simulink model "StereoTypeRobot"  (R2024a)
settings: Solver=VariableStepAuto  StartTime=0.0  StopTime=10.0  RelTol=1e-3
settings Model: Creator=Tamir Azaouag  LastModifiedBy=Tamir Azaouag

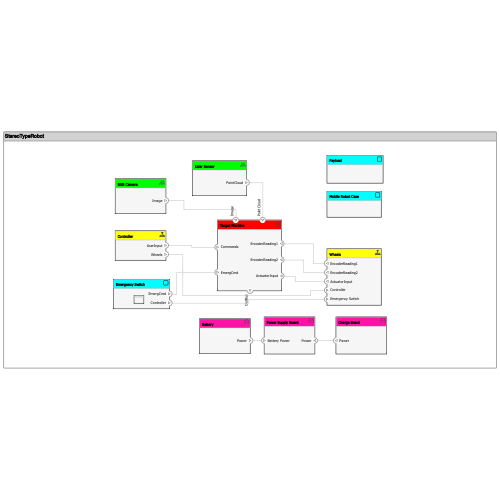
[thumbnail: Simulink's stored preview of the top-level diagram]
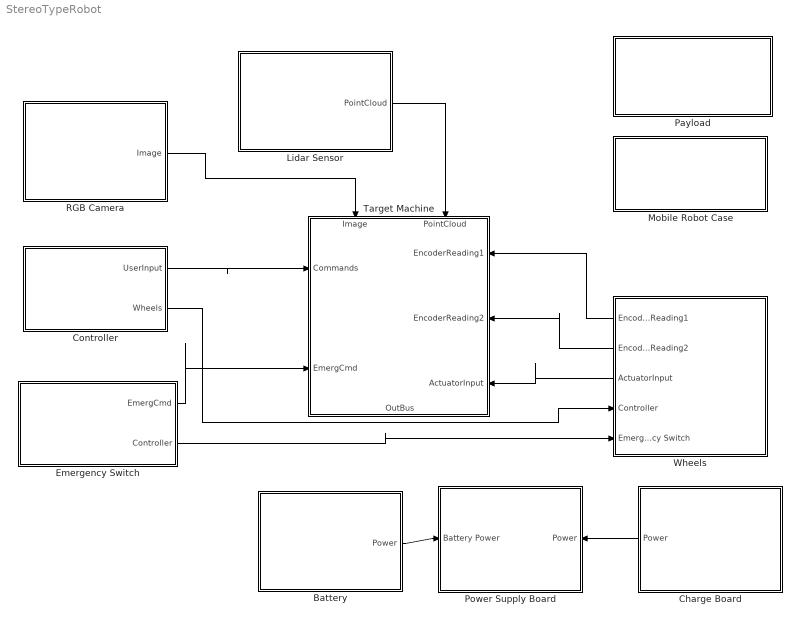
== system StereoTypeRobot ==
  "Battery " : Subsystem
      settings: PortSchema="{\"entries\":[{\"content\":{\"headerSize\":26,\"margin\":15,\"minimumSpacing\":25,\"sides\":[{\"content\":{},\"type\":\"ConnectorPlacement.EquallySpacedRectSide\",\"uuid\":\"52cfc6e8-b07b-405a-8482-438c255d2b0b\"},{\"content\":{\"connectorIds\":[\"Out1\"],\"side\":\"RIGHT\"},\"type\":\"ConnectorPlacement.EquallySpacedRectSide\",\"uuid\":\"f1465f6c-6812-4300-a41b-f67868e7a52d\"},{\"content\":{\"side\":\"TOP\"},\"type\":\"ConnectorPlacement.EquallySpacedRectSide\",\"uuid\":\"9b9722d7-8bd9-4c61-a011-ea6ff4bfa1dc\"}]},\"type\":\"ConnectorPlacement.EquallySpacedConnector\",\"uuid\":\"a33ceaa1-2646-464b-956e-0a789ac4e4be\"}],\"packageUris\":[\"http://schema.mathworks.com/mf0/Connector/R2020b\"],\"version\":\"1.0\"}"
  Charge Board : Subsystem
      settings: PortSchema="{\"entries\":[{\"content\":{\"headerSize\":26,\"margin\":15,\"minimumSpacing\":25,\"sides\":[{\"content\":{\"connectorIds\":[\"Out1\"]},\"type\":\"ConnectorPlacement.EquallySpacedRectSide\",\"uuid\":\"52cfc6e8-b07b-405a-8482-438c255d2b0b\"},{\"content\":{\"side\":\"RIGHT\"},\"type\":\"ConnectorPlacement.EquallySpacedRectSide\",\"uuid\":\"f1465f6c-6812-4300-a41b-f67868e7a52d\"},{\"content\":{\"side\":\"TOP\"},\"type\":\"ConnectorPlacement.EquallySpacedRectSide\",\"uuid\":\"9b9722d7-8bd9-4c61-a011-ea6ff4bfa1dc\"},{\"content\":{\"side\":\"BOTTOM\"},\"type\":\"ConnectorPlacement.EquallySpacedRectSide\",\"uuid\":\"8ae938ba-d761-47b8-bf48-a696c12dfec8\"}]},\"type\":\"ConnectorPlacement.EquallySpacedConnector\",\"uuid\":\"a33ceaa1-2646-464b-956e-0a789ac4e4be\"}],\"packageUris\":[\"http://schema.mathworks.com/mf0/Connector/R2020b\"],\"version\":\"1.0\"}"
  Controller : Subsystem
      settings: PortSchema="{\"entries\":[{\"content\":{\"headerSize\":26,\"margin\":15,\"minimumSpacing\":25,\"sides\":[{\"content\":{},\"type\":\"ConnectorPlacement.EquallySpacedRectSide\",\"uuid\":\"52cfc6e8-b07b-405a-8482-438c255d2b0b\"},{\"content\":{\"connectorIds\":[\"Out1\",\"Out2\"],\"side\":\"RIGHT\"},\"type\":\"ConnectorPlacement.EquallySpacedRectSide\",\"uuid\":\"f1465f6c-6812-4300-a41b-f67868e7a52d\"},{\"content\":{\"side\":\"TOP\"},\"type\":\"ConnectorPlacement.EquallySpacedRectSide\",\"uuid\":\"9b9722d7-8bd9-4c61-a011-ea6ff4bfa1dc\"}]},\"type\":\"ConnectorPlacement.EquallySpacedConnector\",\"uuid\":\"a33ceaa1-2646-464b-956e-0a789ac4e4be\"}],\"packageUris\":[\"http://schema.mathworks.com/mf0/Connector/R2020b\"],\"version\":\"1.0\"}"
  "Emergency Switch " : Subsystem
      settings: PortSchema="{\"entries\":[{\"content\":{\"headerSize\":26,\"margin\":15,\"minimumSpacing\":25,\"sides\":[{\"content\":{},\"type\":\"ConnectorPlacement.EquallySpacedRectSide\",\"uuid\":\"52cfc6e8-b07b-405a-8482-438c255d2b0b\"},{\"content\":{\"connectorIds\":[\"Out1\",\"Out2\"],\"side\":\"RIGHT\"},\"type\":\"ConnectorPlacement.EquallySpacedRectSide\",\"uuid\":\"f1465f6c-6812-4300-a41b-f67868e7a52d\"},{\"content\":{\"side\":\"TOP\"},\"type\":\"ConnectorPlacement.EquallySpacedRectSide\",\"uuid\":\"9b9722d7-8bd9-4c61-a011-ea6ff4bfa1dc\"}]},\"type\":\"ConnectorPlacement.EquallySpacedConnector\",\"uuid\":\"a33ceaa1-2646-464b-956e-0a789ac4e4be\"}],\"packageUris\":[\"http://schema.mathworks.com/mf0/Connector/R2020b\"],\"version\":\"1.0\"}"
  Lidar Sensor : Subsystem
      settings: PortSchema="{\"entries\":[{\"content\":{\"headerSize\":26,\"margin\":15,\"minimumSpacing\":25,\"sides\":[{\"content\":{},\"type\":\"ConnectorPlacement.EquallySpacedRectSide\",\"uuid\":\"52cfc6e8-b07b-405a-8482-438c255d2b0b\"},{\"content\":{\"connectorIds\":[\"Out1\"],\"side\":\"RIGHT\"},\"type\":\"ConnectorPlacement.EquallySpacedRectSide\",\"uuid\":\"f1465f6c-6812-4300-a41b-f67868e7a52d\"},{\"content\":{\"side\":\"TOP\"},\"type\":\"ConnectorPlacement.EquallySpacedRectSide\",\"uuid\":\"9b9722d7-8bd9-4c61-a011-ea6ff4bfa1dc\"}]},\"type\":\"ConnectorPlacement.EquallySpacedConnector\",\"uuid\":\"a33ceaa1-2646-464b-956e-0a789ac4e4be\"}],\"packageUris\":[\"http://schema.mathworks.com/mf0/Connector/R2020b\"],\"version\":\"1.0\"}"
  Mobile Robot Case : Subsystem
      settings: PortSchema="{\"entries\":[{\"content\":{\"headerSize\":26,\"margin\":15,\"minimumSpacing\":25,\"sides\":[{\"content\":{},\"type\":\"ConnectorPlacement.EquallySpacedRectSide\",\"uuid\":\"52cfc6e8-b07b-405a-8482-438c255d2b0b\"},{\"content\":{\"side\":\"RIGHT\"},\"type\":\"ConnectorPlacement.EquallySpacedRectSide\",\"uuid\":\"f1465f6c-6812-4300-a41b-f67868e7a52d\"},{\"content\":{\"side\":\"TOP\"},\"type\":\"ConnectorPlacement.EquallySpacedRectSide\",\"uuid\":\"9b9722d7-8bd9-4c61-a011-ea6ff4bfa1dc\"}]},\"type\":\"ConnectorPlacement.EquallySpacedConnector\",\"uuid\":\"a33ceaa1-2646-464b-956e-0a789ac4e4be\"}],\"packageUris\":[\"http://schema.mathworks.com/mf0/Connector/R2020b\"],\"version\":\"1.0\"}"
  Payload : Subsystem
      settings: PortSchema="{\"entries\":[{\"content\":{\"headerSize\":26,\"margin\":15,\"minimumSpacing\":25,\"sides\":[{\"content\":{},\"type\":\"ConnectorPlacement.EquallySpacedRectSide\",\"uuid\":\"52cfc6e8-b07b-405a-8482-438c255d2b0b\"},{\"content\":{\"side\":\"RIGHT\"},\"type\":\"ConnectorPlacement.EquallySpacedRectSide\",\"uuid\":\"f1465f6c-6812-4300-a41b-f67868e7a52d\"},{\"content\":{\"side\":\"TOP\"},\"type\":\"ConnectorPlacement.EquallySpacedRectSide\",\"uuid\":\"9b9722d7-8bd9-4c61-a011-ea6ff4bfa1dc\"}]},\"type\":\"ConnectorPlacement.EquallySpacedConnector\",\"uuid\":\"a33ceaa1-2646-464b-956e-0a789ac4e4be\"}],\"packageUris\":[\"http://schema.mathworks.com/mf0/Connector/R2020b\"],\"version\":\"1.0\"}"
  Power Supply Board : Subsystem
      settings: PortSchema="{\"entries\":[{\"content\":{\"headerSize\":26,\"margin\":15,\"minimumSpacing\":25,\"sides\":[{\"content\":{\"connectorIds\":[\"In2\"]},\"type\":\"ConnectorPlacement.EquallySpacedRectSide\",\"uuid\":\"52cfc6e8-b07b-405a-8482-438c255d2b0b\"},{\"content\":{\"connectorIds\":[\"In1\"],\"side\":\"RIGHT\"},\"type\":\"ConnectorPlacement.EquallySpacedRectSide\",\"uuid\":\"f1465f6c-6812-4300-a41b-f67868e7a52d\"},{\"content\":{\"side\":\"TOP\"},\"type\":\"ConnectorPlacement.EquallySpacedRectSide\",\"uuid\":\"9b9722d7-8bd9-4c61-a011-ea6ff4bfa1dc\"}]},\"type\":\"ConnectorPlacement.EquallySpacedConnector\",\"uuid\":\"a33ceaa1-2646-464b-956e-0a789ac4e4be\"}],\"packageUris\":[\"http://schema.mathworks.com/mf0/Connector/R2020b\"],\"version\":\"1.0\"}"
  RGB Camera : Subsystem
      settings: PortSchema="{\"entries\":[{\"content\":{\"headerSize\":26,\"margin\":15,\"minimumSpacing\":25,\"sides\":[{\"content\":{},\"type\":\"ConnectorPlacement.EquallySpacedRectSide\",\"uuid\":\"52cfc6e8-b07b-405a-8482-438c255d2b0b\"},{\"content\":{\"connectorIds\":[\"Out1\"],\"side\":\"RIGHT\"},\"type\":\"ConnectorPlacement.EquallySpacedRectSide\",\"uuid\":\"f1465f6c-6812-4300-a41b-f67868e7a52d\"},{\"content\":{\"side\":\"TOP\"},\"type\":\"ConnectorPlacement.EquallySpacedRectSide\",\"uuid\":\"9b9722d7-8bd9-4c61-a011-ea6ff4bfa1dc\"},{\"content\":{\"side\":\"BOTTOM\"},\"type\":\"ConnectorPlacement.EquallySpacedRectSide\",\"uuid\":\"a62c9273-1260-4d0a-a60b-7323b4ab9545\"}]},\"type\":\"ConnectorPlacement.EquallySpacedConnector\",\"uuid\":\"a33ceaa1-2646-464b-956e-0a789ac4e4be\"}],\"packageUris\":[\"http://schema.mathworks.com/mf0/Connector/R2020b\"],\"version\":\"1.0\"}"
  Target Machine : Subsystem
      settings: PortSchema="{\"entries\":[{\"content\":{\"headerSize\":26,\"margin\":15,\"minimumSpacing\":25,\"sides\":[{\"content\":{\"connectorIds\":[\"In6\",\"In7\"]},\"type\":\"ConnectorPlacement.EquallySpacedRectSide\",\"uuid\":\"52cfc6e8-b07b-405a-8482-438c255d2b0b\"},{\"content\":{\"connectorIds\":[\"In1\",\"In2\",\"In3\"],\"side\":\"RIGHT\"},\"type\":\"ConnectorPlacement.EquallySpacedRectSide\",\"uuid\":\"f1465f6c-6812-4300-a41b-f67868e7a52d\"},{\"content\":{\"connectorIds\":[\"In4\",\"In5\"],\"side\":\"TOP\"},\"type\":\"ConnectorPlacement.EquallySpacedRectSide\",\"uuid\":\"9b9722d7-8bd9-4c61-a011-ea6ff4bfa1dc\"},{\"content\":{\"connectorIds\":[\"Out1\"],\"side\":\"BOTTOM\"},\"type\":\"ConnectorPlacement.EquallySpacedRectSide\",\"uuid\":\"d37188e4-ada9-42bd-a53b-1c1899413b13\"}]},\"type\":\"ConnectorPlacement.EquallySpacedConnector\",\"uuid\":\"a33ceaa1-2646-464b-956e-0a789ac4e4be\"}],\"packageUris\":[\"http://schema.mathworks.com/mf0/Connector/R2020b\"],\"version\":\"1.0\"}"
  Wheels : Subsystem
      settings: PortSchema="{\"entries\":[{\"content\":{\"headerSize\":26,\"margin\":15,\"minimumSpacing\":25,\"sides\":[{\"content\":{\"connectorIds\":[\"Out3\",\"Out2\",\"Out1\",\"In1\",\"In2\"]},\"type\":\"ConnectorPlacement.EquallySpacedRectSide\",\"uuid\":\"52cfc6e8-b07b-405a-8482-438c255d2b0b\"},{\"content\":{\"side\":\"RIGHT\"},\"type\":\"ConnectorPlacement.EquallySpacedRectSide\",\"uuid\":\"f1465f6c-6812-4300-a41b-f67868e7a52d\"},{\"content\":{\"side\":\"TOP\"},\"type\":\"ConnectorPlacement.EquallySpacedRectSide\",\"uuid\":\"9b9722d7-8bd9-4c61-a011-ea6ff4bfa1dc\"},{\"content\":{\"side\":\"BOTTOM\"},\"type\":\"ConnectorPlacement.EquallySpacedRectSide\",\"uuid\":\"b29c40a7-1ea8-42d5-9ecb-a2e658638a42\"}]},\"type\":\"ConnectorPlacement.EquallySpacedConnector\",\"uuid\":\"a33ceaa1-2646-464b-956e-0a789ac4e4be\"}],\"packageUris\":[\"http://schema.mathworks.com/mf0/Connector/R2020b\"],\"version\":\"1.0\"}"
  wires:
  "Emergency Switch "/1(EmergCmd) -> Target Machine/7(EmergCmd)
  Controller/1(UserInput) -> Target Machine/6(Commands)
  RGB Camera/1(Image) -> Target Machine/4(Image)
  Lidar Sensor/1(PointCloud) -> Target Machine/5(PointCloud)
  "Battery "/1(Power) -> Power Supply Board/2(Battery Power)
  Charge Board/1(Power) -> Power Supply Board/1(Power)
  Wheels/3(EncoderReading1) -> Target Machine/1(EncoderReading1)
  Wheels/2(EncoderReading2) -> Target Machine/2(EncoderReading2)
  Wheels/1(ActuatorInput) -> Target Machine/3(ActuatorInput)
  Controller/2(Wheels) -> Wheels/1(Controller)
  "Emergency Switch "/2(Controller) -> Wheels/2("Emergency Switch ")

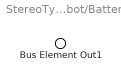
== system StereoTypeRobot/Battery  ==
  Bus Element Out1 : Outport  PortName=Power

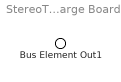
== system StereoTypeRobot/Charge Board ==
  Bus Element Out1 : Outport  PortName=Power

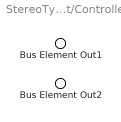
== system StereoTypeRobot/Controller ==
  Bus Element Out1 : Outport  PortName=UserInput
  Bus Element Out2 : Outport  Port=2  PortName=Wheels

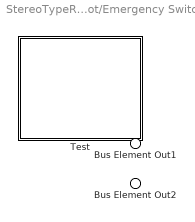
== system StereoTypeRobot/Emergency Switch  ==
  Test : Subsystem
      settings: PortSchema="{\"entries\":[{\"content\":{\"headerSize\":26,\"margin\":15,\"minimumSpacing\":25,\"sides\":[{\"content\":{},\"type\":\"ConnectorPlacement.EquallySpacedRectSide\",\"uuid\":\"a14bca50-eec3-4643-9852-5ab0485d1fad\"},{\"content\":{\"side\":\"RIGHT\"},\"type\":\"ConnectorPlacement.EquallySpacedRectSide\",\"uuid\":\"4c9be622-01ab-4851-b0cd-6570d8f0c0ef\"},{\"content\":{\"side\":\"TOP\"},\"type\":\"ConnectorPlacement.EquallySpacedRectSide\",\"uuid\":\"0b0c369c-b5bb-4b7a-9b2a-cb3d1555d7c6\"}]},\"type\":\"ConnectorPlacement.EquallySpacedConnector\",\"uuid\":\"40fee69b-64dd-44a3-a56b-f30c2048f046\"}],\"packageUris\":[\"http://schema.mathworks.com/mf0/Connector/R2020b\"],\"version\":\"1.0\"}"
  Bus Element Out1 : Outport  PortName=EmergCmd
  Bus Element Out2 : Outport  Port=2  PortName=Controller

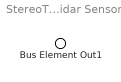
== system StereoTypeRobot/Lidar Sensor ==
  Bus Element Out1 : Outport  PortName=PointCloud

== system StereoTypeRobot/Mobile Robot Case ==

== system StereoTypeRobot/Payload ==

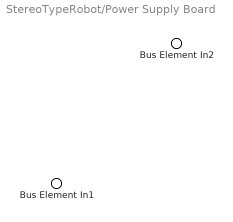
== system StereoTypeRobot/Power Supply Board ==
  Bus Element In2 : Inport  PortName=Power
  Bus Element In1 : Inport  Port=2  PortName=Battery Power

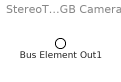
== system StereoTypeRobot/RGB Camera ==
  Bus Element Out1 : Outport  PortName=Image

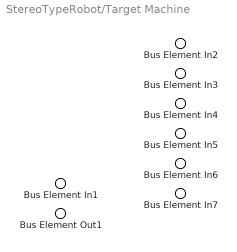
== system StereoTypeRobot/Target Machine ==
  Bus Element In5 : Inport  PortName=EncoderReading1
  Bus Element In6 : Inport  Port=2  PortName=EncoderReading2
  Bus Element In7 : Inport  Port=3  PortName=ActuatorInput
  Bus Element In3 : Inport  Port=4  PortName=Image
  Bus Element In4 : Inport  Port=5  PortName=PointCloud
  Bus Element In2 : Inport  Port=6  PortName=Commands
  Bus Element In1 : Inport  Port=7  PortName=EmergCmd
  Bus Element Out1 : Outport  PortName=OutBus

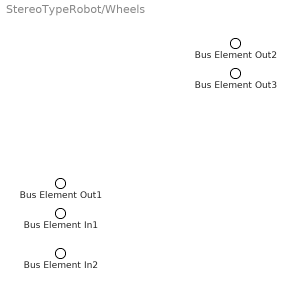
== system StereoTypeRobot/Wheels ==
  Bus Element In1 : Inport  PortName=Controller
  Bus Element In2 : Inport  Port=2  PortName=Emergency Switch
  Bus Element Out3 : Outport  PortName=ActuatorInput
  Bus Element Out2 : Outport  Port=2  PortName=EncoderReading2
  Bus Element Out1 : Outport  Port=3  PortName=EncoderReading1

== system StereoTypeRobot/Emergency Switch /Test ==
